simulink model "Lab1PartC52"  (R2023b)
settings: Solver=VariableStepAuto  StartTime=0.0  StopTime=10  RelTol=1e-3
settings Model: Creator=m96sz  LastModifiedBy=m96sz

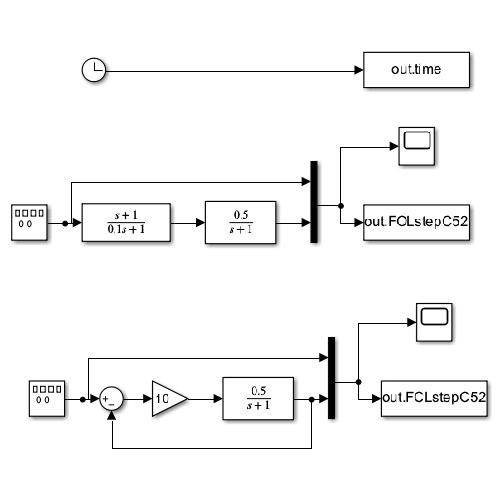
[thumbnail: Simulink's stored preview of the top-level diagram]
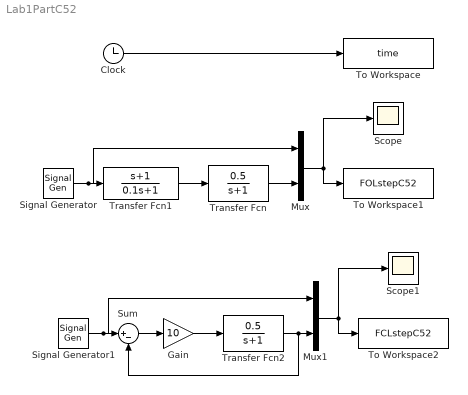
== system Lab1PartC52 ==
  Clock : Clock
      settings: Decimation=100
  Gain : Gain  Gain=10
  Mux : Mux  Inputs=2
  Mux1 : Mux  Inputs=2
  Scope : Scope
  Scope1 : Scope
  Signal Generator : SignalGenerator  WaveForm=square  Frequency=0.25
  Signal Generator1 : SignalGenerator  WaveForm=square  Frequency=0.25
  Sum : Sum  Inputs=|+-
  To Workspace : ToWorkspace  VariableName=time  SampleTime=-1
  To Workspace1 : ToWorkspace  VariableName=FOLstepC52  SampleTime=-1
  To Workspace2 : ToWorkspace  VariableName=FCLstepC52  SampleTime=-1
  Transfer Fcn : TransferFcn  Numerator=[0.5]  Denominator=[1 1]
  Transfer Fcn1 : TransferFcn  Numerator=[1 1]  Denominator=[0.1 1]
  Transfer Fcn2 : TransferFcn  Numerator=[0.5]  Denominator=[1 1]
  wires:
  Transfer Fcn/1 -> Mux/2
  Clock/1 -> To Workspace/1
  Mux/1 -> To Workspace1/1, Scope/1
  Transfer Fcn1/1 -> Transfer Fcn/1
  Signal Generator/1 -> Mux/1, Transfer Fcn1/1
  Transfer Fcn2/1 -> Sum/2, Mux1/2
  Signal Generator1/1 -> Mux1/1, Sum/1
  Mux1/1 -> To Workspace2/1, Scope1/1
  Sum/1 -> Gain/1
  Gain/1 -> Transfer Fcn2/1
